simulink model "flyback_ideal"  (R2023b)
settings: Solver=VariableStepAuto  StartTime=0.0  StopTime=0.001  RelTol=1e-3
libraries: spsSeriesRLCBranchLib x2, spsVoltageMeasurementLib x2, spsDCVoltageSourceLib x1, spsCurrentMeasurementLib x1, spsDiodeLib x1, spsLinearTransformerLib x1, spsMosfetLib x1, spsRMSLib x1, sps_lib x1
settings Model: Creator=Msi  LastModifiedBy=Msi

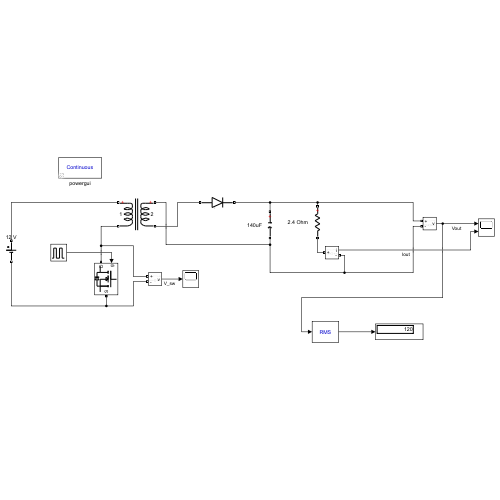
[thumbnail: Simulink's stored preview of the top-level diagram]
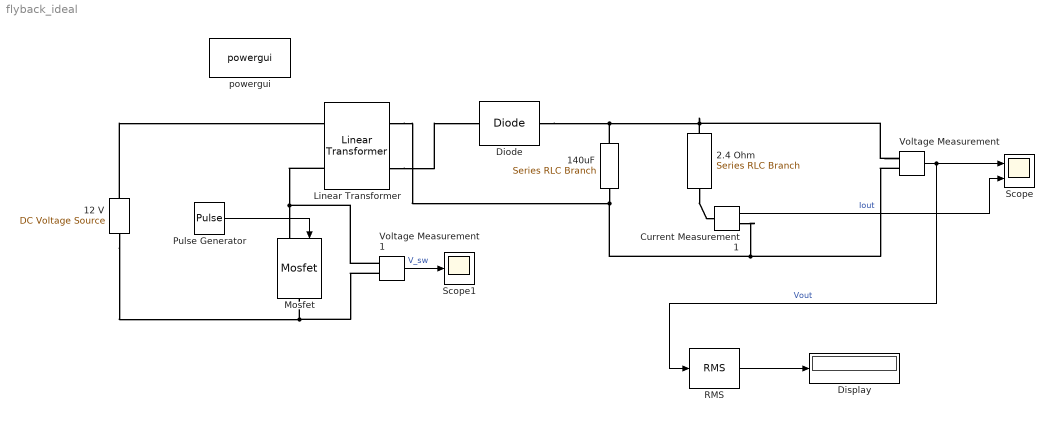
== system flyback_ideal ==
  12 V : spsDCVoltageSourceLib/DC Voltage Source  Amplitude=40  Measurements=None
  140uF : spsSeriesRLCBranchLib/Series RLC Branch  LConnTagsString=__new0  RConnTagsString=__new0  BranchType=C  Resistance=1  Inductance=1e-3  SetiL0=off  InitialCurrent=0  Capacitance=140e-6  Setx0=off  InitialVoltage=0  Measurements=None
  2.4 Ohm : spsSeriesRLCBranchLib/Series RLC Branch  LConnTagsString=__new0  RConnTagsString=__new0  BranchType=R  Resistance=12/5  Inductance=1e-3  SetiL0=off  InitialCurrent=0  Capacitance=1e-6  Setx0=off  InitialVoltage=0  Measurements=None
  Current Measurement1 : spsCurrentMeasurementLib/Current Measurement  PhasorSimulation=off  OutputType=Complex  PSBequivalent=0
  Diode : spsDiodeLib/Diode  Ron=0.001  Lon=0  Vf=0  IC=0  UseSnubber=0  Rs=0  Cs=0  Measurements=off
  Display : Display
  Linear Transformer : spsLinearTransformerLib/Linear Transformer  UNITS=SI  NominalPower=[ 100 100e3 ]  winding1=[20 0 0]  winding2=[10 0 0]  ThreeWindings=off  winding3=[3.15e+05 0.7938 0.084225]  RmLm=[1 26e-6]  Measurements=None  DataType=on
  Mosfet : spsMosfetLib/Mosfet  Ron=0  Lon=0  Rd=0  Vfd=0  IC=0  Rs=1e5  Cs=inf  Measurements=off
  Pulse Generator : DiscretePulseGenerator  PulseType=Time based  Period=1/(100e3)  PulseWidth=37.6
  RMS : spsRMSLib/RMS  TrueRMS=on  Freq=60  RMSInit=120  Ts=0
  Scope : Scope  NumInputPorts=2
  Scope1 : Scope
  Voltage Measurement : spsVoltageMeasurementLib/Voltage Measurement  PhasorSimulation=off  OutputType=Complex  PSBequivalent=0
  Voltage Measurement1 : spsVoltageMeasurementLib/Voltage Measurement  PhasorSimulation=off  OutputType=Complex  PSBequivalent=0
  powergui : sps_lib/powergui  Priority=1  SimulationMode=Continuous  SampleTime=50e-6  frequency=60  Iterations=50  frequencyindice=0  Pbase=100e6  ErrMax=1e-4  UnitsV=kV  UnitsW=MW  buscounter=0  FunctionMessages=off  echomessages=off  EnableUseOfTLC=off  CurrentSourceSwitches=off  DisableSnubberDevices=off  DisableRonSwitches=off  DisableVfSwitches=off  DisplayEquations=off  AutomaticDiscreteSolvers=off  SolverType=Tustin/Backward Euler (TBE)  Interpol=off  ExternalGateDelay=off  methode=off  Ts=100  x0status=blocks  SPID=on  SwTol=0  HookPort=off  NonlinearTolerance=1e-4  nMaxIteration=100  ContinueOnMaxIteration=off  RestoreLinks=warning  ResistiveCurrentMeasurement=off  Frange=[0:2:500]  Ylog=off  Xlog=on  ShowGrid=off  save=off  variable=ZData  structure=0  ZoomFFT=off  StartTime=0.0  cycles=1  DisplayStyle=1  fundamental=60  FreqAxis=off  MaxFrequency=1000  frequencyindicesteady=1  RmsSteady=1  display=off
  wires:
  Voltage Measurement/1 -> RMS/1, Scope/1  "Vout"
  RMS/1 -> Display/1
  Pulse Generator/1 -> Mosfet/1
  Current Measurement1/1 -> Scope/2  "Iout"
  Voltage Measurement1/1 -> Scope1/1  "V_sw"
  connections:
  Linear Transformer/LConn2 -- Voltage Measurement1/LConn1 -- Mosfet/LConn1
  12 V/RConn1 -- Linear Transformer/LConn1
  Linear Transformer/RConn1 -- Current Measurement1/RConn1 -- Voltage Measurement/LConn2 -- 140uF/RConn1
  2.4 Ohm/LConn1 -- Diode/RConn1 -- 140uF/LConn1 -- Voltage Measurement/LConn1
  Linear Transformer/RConn2 -- Diode/LConn1
  Voltage Measurement1/LConn2 -- 12 V/LConn1 -- Mosfet/RConn1
  2.4 Ohm/RConn1 -- Current Measurement1/LConn1
